simulink model "BG"  (R2014a)
settings: Solver=FixedStepDiscrete  StartTime=0.0  StopTime=24  FixedStep=dt  RelTol=1e-3
values from neighbouring files (symbols this model uses):
  a1 = 5    [parameters.m]
  a2 = 3    [parameters.m]
  a3 = 2    [parameters.m]
  delay = 1    [parameters.m]
  dt = 1e-3    (= 0.001)    [parameters.m]
  g = 1    [parameters.m]
  OP1_0 = [ax1_0 ay1_0 0]    [parameters.m]
  OP2_0 = OP1_0 + P1P2_0    [parameters.m]
  OP3_0 = OP2_0 + P2P3_0    [parameters.m]
  OT1 = [4 6 0]    [animation.m]    (also in parameters.m)
  OT10 = [-1 7.5 0]    [parameters.m]
  OT11 = [3 4.5 0]    [parameters.m]
  OT12 = [-1 7.5 0]    [parameters.m]
  OT2 = [-2 6 0]    [animation.m]    (also in parameters.m)
  OT3 = [1 8 0]    [animation.m]    (also in parameters.m = [4 6 0])
  OT4 = [1 4 0]    [animation.m]    (also in parameters.m = [1 8 0])
  OT5 = [3 7.5 0]    [animation.m]    (also in parameters.m = [1 4 0])
  OT6 = [-1 4.5 0]    [animation.m]    (also in parameters.m = [1 8 0])
  OT7 = [-1 7.5 0]    [animation.m]    (also in parameters.m = [3 7.5 0])
  OT8 = [3 4.5 0]    [animation.m]    (also in parameters.m = [-1 4.5 0])
  OT9 = [3 7.5 0]    [parameters.m]
  P1P2_0 = [ax2_0 ay2_0 0]    [parameters.m]
  P2P3_0 = [ax3_0 ay3_0 0]    [parameters.m]
  w1 = 1/100    (= 0.01)    [parameters.m]
  w2 = 1/50    (= 0.02)    [parameters.m]
  w3 = 1/20    (= 0.05)    [parameters.m]
  zero_vector = [0 0 0]    [parameters.m]
libraries: vrlib x6, simulink x1
settings Model: Creator=Armin  LastModifiedBy=Armin

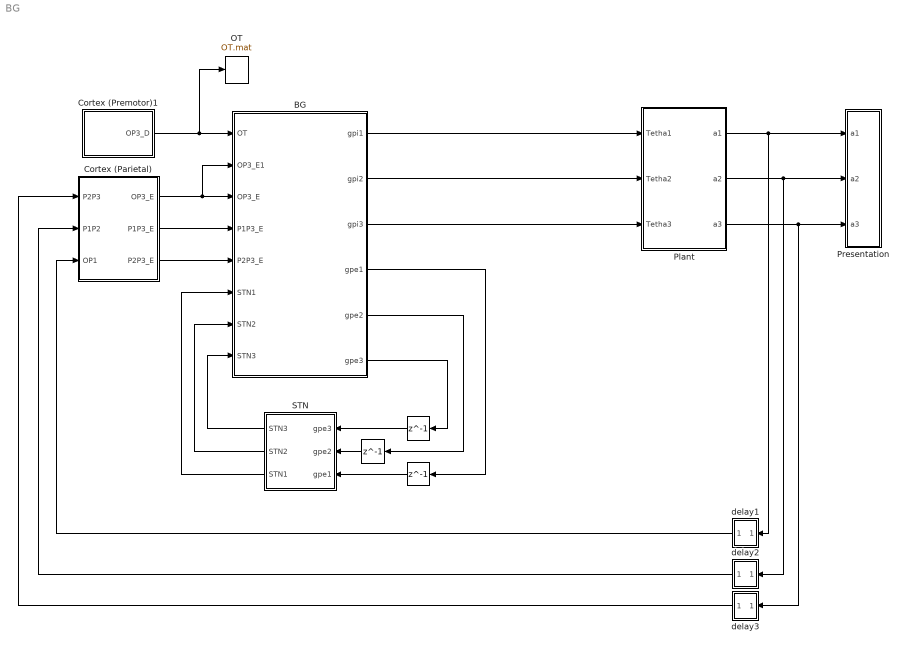
== system BG ==
  "                    " : Delay  DelayLength=1  InitialCondition=zero_vector
  "                     " : Delay  DelayLength=1  InitialCondition=zero_vector
  "                      " : Delay  DelayLength=1  InitialCondition=zero_vector
  BG : Subsystem
  Cortex (Parietal) : Subsystem
  Cortex (Premotor)1 : Subsystem
  OT : ToFile  Filename=OT.mat  MatrixName=T
  Plant : Subsystem
  Presentation : Subsystem
  STN : Subsystem
  delay1 : Subsystem
  delay2 : Subsystem
  delay3 : Subsystem
  wires:
  Plant/1(a1) -> Presentation/1(a1), delay1/1(In1)
  Plant/2(a2) -> Presentation/2(a2), delay2/1(In1)
  BG/1(gpi1) -> Plant/1(Tetha1)
  BG/2(gpi2) -> Plant/2(Tetha2)
  delay2/1(Out1) -> Cortex (Parietal)/2(P1P2)
  delay1/1(Out1) -> Cortex (Parietal)/3(OP1)
  Cortex (Parietal)/1(OP3_E) -> BG/2(OP3_E1), BG/3(OP3_E)
  Cortex (Parietal)/2(P1P3_E) -> BG/4(P1P3_E)
  Cortex (Parietal)/3(P2P3_E) -> BG/5(P2P3_E)
  BG/3(gpi3) -> Plant/3(Tetha3)
  Plant/3(a3) -> Presentation/3(a3), delay3/1(In1)
  delay3/1(Out1) -> Cortex (Parietal)/1(P2P3)
  BG/6(gpe3) -> "                    "/1
  BG/5(gpe2) -> "                     "/1
  BG/4(gpe1) -> "                      "/1
  "                    "/1 -> STN/1(gpe3)
  "                     "/1 -> STN/2(gpe2)
  "                      "/1 -> STN/3(gpe1)
  STN/3(STN1) -> BG/6(STN1)
  STN/2(STN2) -> BG/7(STN2)
  STN/1(STN3) -> BG/8(STN3)
  Cortex (Premotor)1/1(OP3_D) -> OT/1, BG/1(OT)

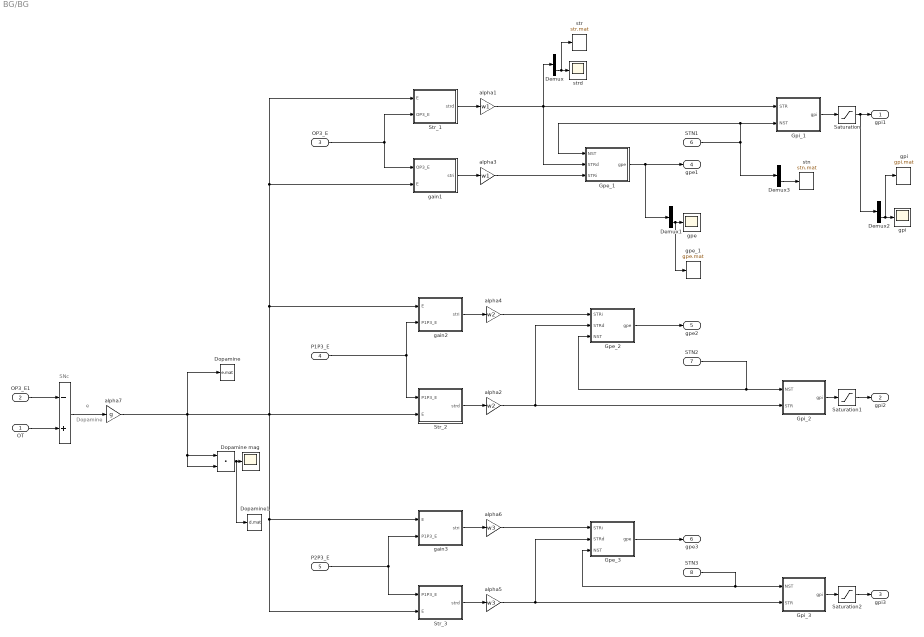
== system BG/BG ==
  note: Dopamine
  note: e
  note: SNc
  OT : Inport
  OP3_E1 : Inport  Port=2
  OP3_E : Inport  Port=3
  P1P3_E : Inport  Port=4
  P2P3_E : Inport  Port=5
  STN1 : Inport  Port=6
  STN2 : Inport  Port=7
  STN3 : Inport  Port=8
  " " : Sum  Inputs=-+
  "     " : DotProduct  InputSameDT=on  OutDataTypeStr=Inherit: Inherit via internal rule
  Demux{,1..3} (4 alike) : Demux  Outputs=3
  Dopamine : ToFile  Filename=e.mat  MatrixName=e
  Dopamine mag : Scope
      settings: SaveName=ScopeData7
  Dopamine1 : ToFile  Filename=d.mat  MatrixName=d
  Gpe_1 : Subsystem
  Gpe_2 : Subsystem
  Gpe_3 : Subsystem
  Gpi_1 : Subsystem
  Gpi_2 : Subsystem
  Gpi_3 : Subsystem
  Saturation : Saturate  UpperLimit=pi  LowerLimit=-pi
  Saturation1 : Saturate  UpperLimit=pi  LowerLimit=-pi
  Saturation2 : Saturate  UpperLimit=pi  LowerLimit=-pi
  Str_1 : Subsystem
  Str_2 : Subsystem
  Str_3 : Subsystem
  alpha1 : Gain  Gain=w1
  alpha2 : Gain  Gain=w2
  alpha3 : Gain  Gain=w1
  alpha4 : Gain  Gain=w2
  alpha5 : Gain  Gain=w3
  alpha6 : Gain  Gain=w3
  alpha7 : Gain  Gain=g
  gain1 : Subsystem
  gain2 : Subsystem
  gain3 : Subsystem
  gpe : Scope
      settings: SaveName=ScopeData5
  gpe_1 : ToFile  Filename=gpe.mat  MatrixName=gpe
  gpi : Scope
      settings: SaveName=ScopeData6
  "gpi " : ToFile  Filename=gpi.mat  MatrixName=gpi
  stn : ToFile  Filename=stn.mat  MatrixName=stn
  str : ToFile  Filename=str.mat  MatrixName=str
  strd : Scope
  gpi1 : Outport
  gpi2 : Outport  Port=2
  gpi3 : Outport  Port=3
  gpe1 : Outport  Port=4
  gpe2 : Outport  Port=5
  gpe3 : Outport  Port=6
  wires:
  Str_1/1(strd) -> alpha1/1
  OP3_E/1 -> gain1/1(OP3_E), Str_1/2(OP3_E)
  Str_2/1(strd) -> alpha2/1
  gain1/1(stri) -> alpha3/1
  alpha3/1 -> Gpe_1/3(STRi)
  Gpe_1/1(gpe) -> Demux1/1, gpe1/1
  STN1/1 -> Demux3/1, Gpi_1/2(NST), Gpe_1/1(NST)
  gain2/1(stri) -> alpha4/1
  alpha4/1 -> Gpe_2/1(STRi)
  P1P3_E/1 -> Str_2/1(P1P3_E), gain2/2(P1P3_E)
  Gpe_2/1(gpe) -> gpe2/1
  OT/1 -> " "/2
  Str_3/1(strd) -> alpha5/1
  gain3/1(stri) -> alpha6/1
  alpha6/1 -> Gpe_3/1(STRi)
  P2P3_E/1 -> Str_3/1(P1P3_E), gain3/2(P1P3_E)
  Gpe_3/1(gpe) -> gpe3/1
  " "/1 -> alpha7/1
  OP3_E1/1 -> " "/1
  Gpi_2/1(gpi) -> Saturation1/1
  Gpi_3/1(gpi) -> Saturation2/1
  Demux/3 -> str/1, strd/1
  Demux1/3 -> gpe_1/1, gpe/1
  Gpi_1/1(gpi) -> Saturation/1
  Demux2/3 -> "gpi "/1, gpi/1
  STN3/1 -> Gpi_3/1(NST), Gpe_3/3(NST)
  STN2/1 -> Gpi_2/1(NST), Gpe_2/3(NST)
  alpha1/1 -> Gpi_1/1(STR), Demux/1, Gpe_1/2(STRd)
  alpha2/1 -> Gpi_2/2(STR), Gpe_2/2(STRd)
  alpha5/1 -> Gpi_3/2(STR), Gpe_3/2(STRd)
  "     "/1 -> Dopamine1/1, Dopamine mag/1
  alpha7/1 -> Str_1/1(E), gain1/2(E), gain2/1(E), Str_2/2(E), gain3/1(E), Str_3/2(E), Dopamine/1, "     "/1, "     "/2
  Saturation/1 -> Demux2/1, gpi1/1
  Saturation1/1 -> gpi2/1
  Saturation2/1 -> gpi3/1
  Demux3/3 -> stn/1

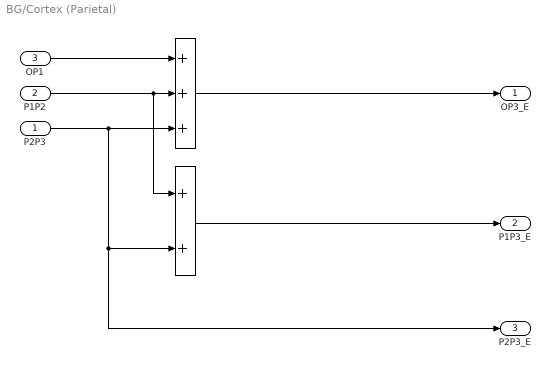
== system BG/Cortex (Parietal) ==
  P2P3 : Inport
  P1P2 : Inport  Port=2
  OP1 : Inport  Port=3
  " " : Sum  Inputs=+++
  "  " : Sum
  OP3_E : Outport
  P1P3_E : Outport  Port=2
  P2P3_E : Outport  Port=3
  wires:
  OP1/1 -> " "/1
  P1P2/1 -> "  "/1, " "/2
  P2P3/1 -> P2P3_E/1, "  "/2, " "/3
  " "/1 -> OP3_E/1
  "  "/1 -> P1P3_E/1

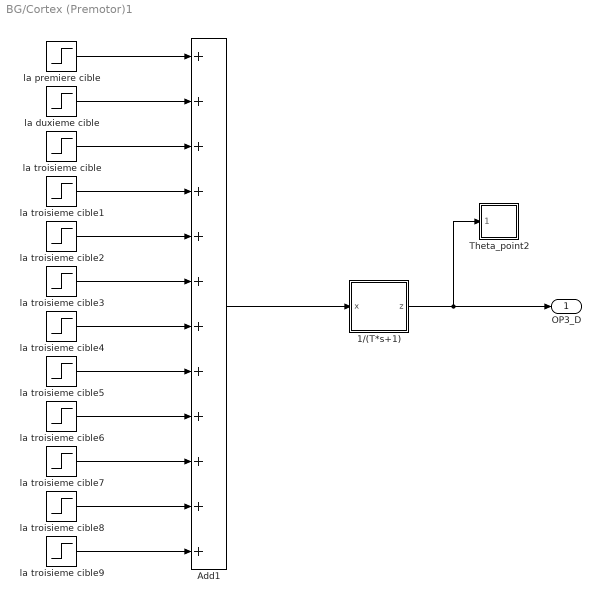
== system BG/Cortex (Premotor)1 ==
  1/(T*s+1) : Subsystem  TreatAsAtomicUnit=on
  Add1 : Sum  Inputs=++++++++++++
  Theta_point2 : Subsystem
  la duxieme cible : Step  Time=2  After=OT2-OT1  SampleTime=0
  la premiere cible : Step  Time=0.05  Before=OP3_0  After=OT1  SampleTime=0
  la troisieme cible : Step  Time=4  After=OT3-OT2  SampleTime=0
  la troisieme cible1 : Step  Time=6  After=OT4-OT3  SampleTime=0
  la troisieme cible2 : Step  Time=8  After=OT5-OT4  SampleTime=0
  la troisieme cible3 : Step  Time=10  After=OT6-OT5  SampleTime=0
  la troisieme cible4 : Step  Time=12  After=OT7-OT6  SampleTime=0
  la troisieme cible5 : Step  Time=14  After=OT8-OT7  SampleTime=0
  la troisieme cible6 : Step  Time=16  After=OT9-OT8  SampleTime=0
  la troisieme cible7 : Step  Time=18  After=OT10-OT9  SampleTime=0
  la troisieme cible8 : Step  Time=20  After=OT11-OT10  SampleTime=0
  la troisieme cible9 : Step  Time=22  After=OT12-OT11  SampleTime=0
  OP3_D : Outport
  wires:
  1/(T*s+1)/1(z) -> Theta_point2/1(In_vec), OP3_D/1
  Add1/1 -> 1/(T*s+1)/1(x)
  la premiere cible/1 -> Add1/1
  la duxieme cible/1 -> Add1/2
  la troisieme cible/1 -> Add1/3
  la troisieme cible1/1 -> Add1/4
  la troisieme cible2/1 -> Add1/5
  la troisieme cible3/1 -> Add1/6
  la troisieme cible4/1 -> Add1/7
  la troisieme cible5/1 -> Add1/8
  la troisieme cible6/1 -> Add1/9
  la troisieme cible7/1 -> Add1/10
  la troisieme cible8/1 -> Add1/11
  la troisieme cible9/1 -> Add1/12

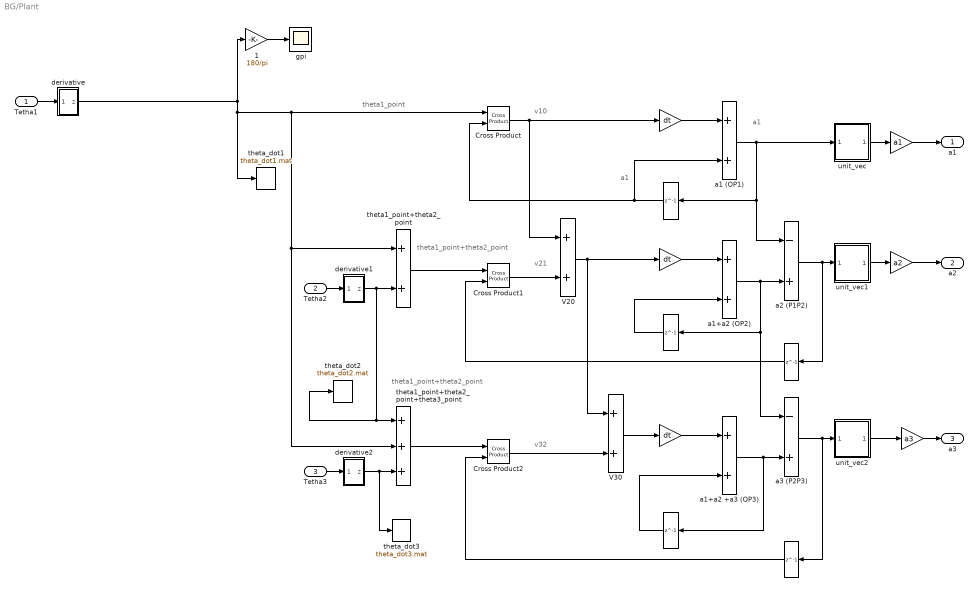
== system BG/Plant ==
  note: theta1_point
  note: a1
  note: v10
  note: a1
  note: theta1_point+theta2_point
  note: v21
  note: theta1_point+theta2_point
  note: v32
  Tetha1 : Inport
  Tetha2 : Inport  Port=2
  Tetha3 : Inport  Port=3
  " " : Delay  DelayLength=1  InitialCondition=OP1_0
  "  " : Delay  DelayLength=1  InitialCondition=OP2_0
  "        " : Gain  Gain=dt
  "         " : Gain  Gain=a1
  "          " : Delay  DelayLength=1  InitialCondition=OP3_0
  "              " : Gain  Gain=a2
  "                  " : Delay  DelayLength=1  InitialCondition=P1P2_0
  "                         " : Gain  Gain=a3
  "                                  " : Gain  Gain=dt
  "                                                             " : Gain  Gain=dt
  "                                                              " : Delay  DelayLength=1  InitialCondition=P2P3_0
  "        1" : Gain  Gain=180/pi
  "Cross Product " : vrlib/Utilities/Cross Product
  Cross Product1 : vrlib/Utilities/Cross Product
  Cross Product2 : vrlib/Utilities/Cross Product
  V20 : Sum
  V30 : Sum
  a1 (OP1) : Sum
  a1+a2 (OP2) : Sum
  a1+a2 +a3 (OP3) : Sum
  a2 (P1P2) : Sum  Inputs=-+
  a3 (P2P3) : Sum  Inputs=-+
  derivative : Subsystem  TreatAsAtomicUnit=on
  derivative1 : Subsystem  TreatAsAtomicUnit=on
  derivative2 : Subsystem  TreatAsAtomicUnit=on
  gpi : Scope
      settings: YMin=-6.5e-35  YMax=0  SaveName=ScopeData8
  theta1_point+theta2_point : Sum
  theta1_point+theta2_point+theta3_point : Sum  Inputs=+++
  theta_dot1 : ToFile  Filename=theta_dot1.mat  MatrixName=theta_dot1
  theta_dot2 : ToFile  Filename=theta_dot2.mat  MatrixName=theta_dot2
  theta_dot3 : ToFile  Filename=theta_dot3.mat  MatrixName=theta_dot3
  unit_vec : Subsystem
  unit_vec1 : Subsystem
  unit_vec2 : Subsystem
  a1 : Outport
  a2 : Outport  Port=2
  a3 : Outport  Port=3
  wires:
  "        "/1 -> a1 (OP1)/1
  " "/1 -> "Cross Product "/2, a1 (OP1)/2
  Tetha1/1 -> derivative/1(x)
  Tetha2/1 -> derivative1/1(x)
  theta1_point+theta2_point/1 -> Cross Product1/1
  Tetha3/1 -> derivative2/1(x)
  theta1_point+theta2_point+theta3_point/1 -> Cross Product2/1
  V20/1 -> "                                  "/1, V30/1
  "                                  "/1 -> a1+a2 (OP2)/1
  a1+a2 (OP2)/1 -> a2 (P1P2)/2, a3 (P2P3)/1, "  "/1
  "  "/1 -> a1+a2 (OP2)/2
  "                  "/1 -> Cross Product1/2
  V30/1 -> "                                                             "/1
  a1+a2 +a3 (OP3)/1 -> a3 (P2P3)/2, "          "/1
  "          "/1 -> a1+a2 +a3 (OP3)/2
  "                                                              "/1 -> Cross Product2/2
  "                                                             "/1 -> a1+a2 +a3 (OP3)/1
  "Cross Product "/1 -> V20/1, "        "/1
  Cross Product1/1 -> V20/2
  Cross Product2/1 -> V30/2
  a1 (OP1)/1 -> a2 (P1P2)/1, " "/1, unit_vec/1(vec1)
  a2 (P1P2)/1 -> "                  "/1, unit_vec1/1(vec1)
  a3 (P2P3)/1 -> unit_vec2/1(vec1), "                                                              "/1
  unit_vec/1(vec2) -> "         "/1
  "         "/1 -> a1/1
  unit_vec1/1(vec2) -> "              "/1
  "              "/1 -> a2/1
  "                         "/1 -> a3/1
  unit_vec2/1(vec2) -> "                         "/1
  derivative1/1(z) -> theta_dot2/1, theta1_point+theta2_point+theta3_point/1, theta1_point+theta2_point/2
  derivative2/1(z) -> theta_dot3/1, theta1_point+theta2_point+theta3_point/3
  "        1"/1 -> gpi/1
  derivative/1(z) -> theta_dot1/1, "Cross Product "/1, theta1_point+theta2_point/1, theta1_point+theta2_point+theta3_point/2, "        1"/1

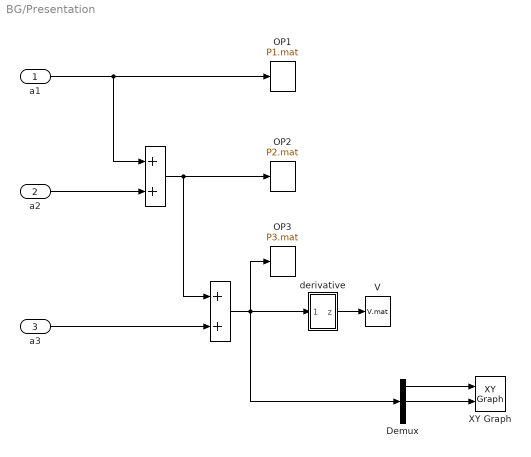
== system BG/Presentation ==
  a1 : Inport
  a2 : Inport  Port=2
  a3 : Inport  Port=3
  "                       " : Sum
  "                        " : Sum
  Demux : Demux  Outputs=3
  OP1 : ToFile  Filename=P1.mat  MatrixName=P1
  OP2 : ToFile  Filename=P2.mat  MatrixName=P2
  OP3 : ToFile  Filename=P3.mat  MatrixName=P3
  V : ToFile  Filename=V.mat  MatrixName=V
  XY Graph : simulink/Sinks/XY Graph  xmin=-10  xmax=10  ymin=0  ymax=10  st=-1
  derivative : Subsystem  TreatAsAtomicUnit=on
  wires:
  a1/1 -> "                       "/1, OP1/1
  a2/1 -> "                       "/2
  "                       "/1 -> "                        "/1, OP2/1
  a3/1 -> "                        "/2
  "                        "/1 -> Demux/1, OP3/1, derivative/1(x)
  derivative/1(z) -> V/1
  Demux/1 -> XY Graph/1
  Demux/2 -> XY Graph/2

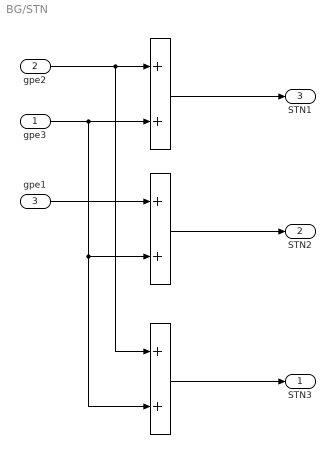
== system BG/STN ==
  gpe3 : Inport
  gpe2 : Inport  Port=2
  gpe1 : Inport  Port=3
  " " : Sum
  "  " : Sum
  "    " : Sum
  STN3 : Outport
  STN2 : Outport  Port=2
  STN1 : Outport  Port=3
  wires:
  " "/1 -> STN1/1
  gpe3/1 -> " "/2, "    "/2, "  "/2
  gpe2/1 -> " "/1, "    "/1
  "  "/1 -> STN2/1
  gpe1/1 -> "  "/1
  "    "/1 -> STN3/1

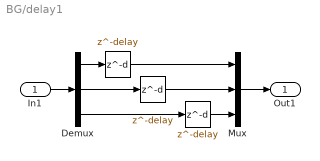
== system BG/delay1 ==
  In1 : Inport
  "  " : Delay  DelayLength=delay  InitialCondition=OP1_0(2)
  "   " : Delay  DelayLength=delay  InitialCondition=OP1_0(3)
  "                                                                                                                                               \t" : Delay  DelayLength=delay  InitialCondition=OP1_0(1)
  Demux : Demux  Outputs=3
  Mux : Mux  Inputs=3
  Out1 : Outport
  wires:
  Mux/1 -> Out1/1
  In1/1 -> Demux/1
  "                                                                                                                                               \t"/1 -> Mux/1
  Demux/1 -> "                                                                                                                                               \t"/1
  "  "/1 -> Mux/2
  Demux/2 -> "  "/1
  "   "/1 -> Mux/3
  Demux/3 -> "   "/1

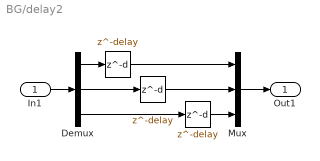
== system BG/delay2 ==
  In1 : Inport
  "  " : Delay  DelayLength=delay  InitialCondition=P1P2_0(2)
  "   " : Delay  DelayLength=delay  InitialCondition=P1P2_0(3)
  "                                                                                                                                               \t" : Delay  DelayLength=delay  InitialCondition=P1P2_0(1)
  Demux : Demux  Outputs=3
  Mux : Mux  Inputs=3
  Out1 : Outport
  wires:
  Mux/1 -> Out1/1
  In1/1 -> Demux/1
  "                                                                                                                                               \t"/1 -> Mux/1
  Demux/1 -> "                                                                                                                                               \t"/1
  "  "/1 -> Mux/2
  Demux/2 -> "  "/1
  "   "/1 -> Mux/3
  Demux/3 -> "   "/1

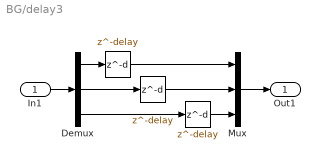
== system BG/delay3 ==
  In1 : Inport
  "  " : Delay  DelayLength=delay  InitialCondition=P2P3_0(2)
  "   " : Delay  DelayLength=delay  InitialCondition=P2P3_0(3)
  "                                                                                                                                               \t" : Delay  DelayLength=delay  InitialCondition=P2P3_0(1)
  Demux : Demux  Outputs=3
  Mux : Mux  Inputs=3
  Out1 : Outport
  wires:
  Mux/1 -> Out1/1
  In1/1 -> Demux/1
  "                                                                                                                                               \t"/1 -> Mux/1
  Demux/1 -> "                                                                                                                                               \t"/1
  "  "/1 -> Mux/2
  Demux/2 -> "  "/1
  "   "/1 -> Mux/3
  Demux/3 -> "   "/1

== system BG/BG/Gpe_1 ==
  NST : Inport
  STRd : Inport  Port=2
  STRi : Inport  Port=3
  "   " : Product
  GPi1 : Sum  Inputs=+-
  gpe : Outport
  wires:
  STRd/1 -> GPi1/1
  NST/1 -> GPi1/2
  GPi1/1 -> "   "/1
  STRi/1 -> "   "/2
  "   "/1 -> gpe/1

== system BG/BG/Gpe_2 ==
  STRi : Inport
  STRd : Inport  Port=2
  NST : Inport  Port=3
  "   " : Product
  GPi1 : Sum  Inputs=+-
  gpe : Outport
  wires:
  STRd/1 -> GPi1/1
  NST/1 -> GPi1/2
  GPi1/1 -> "   "/1
  STRi/1 -> "   "/2
  "   "/1 -> gpe/1

== system BG/BG/Gpe_3 ==
  STRi : Inport
  STRd : Inport  Port=2
  NST : Inport  Port=3
  "   " : Product
  GPi1 : Sum  Inputs=+-
  gpe : Outport
  wires:
  STRd/1 -> GPi1/1
  NST/1 -> GPi1/2
  GPi1/1 -> "   "/1
  STRi/1 -> "   "/2
  "   "/1 -> gpe/1

== system BG/BG/Gpi_1 ==
  STR : Inport
  NST : Inport  Port=2
  "                  " : Delay  DelayLength=1  InitialCondition=zero_vector
  GPi1 : Sum  Inputs=++-
  gpi : Outport
  wires:
  GPi1/1 -> "                  "/1, gpi/1
  "                  "/1 -> GPi1/1
  STR/1 -> GPi1/2
  NST/1 -> GPi1/3

== system BG/BG/Gpi_2 ==
  NST : Inport
  STR : Inport  Port=2
  "                  " : Delay  DelayLength=1  InitialCondition=zero_vector
  GPi1 : Sum  Inputs=++-
  gpi : Outport
  wires:
  GPi1/1 -> "                  "/1, gpi/1
  "                  "/1 -> GPi1/1
  STR/1 -> GPi1/2
  NST/1 -> GPi1/3

== system BG/BG/Gpi_3 ==
  NST : Inport
  STR : Inport  Port=2
  "                  " : Delay  DelayLength=1  InitialCondition=zero_vector
  GPi1 : Sum  Inputs=++-
  gpi : Outport
  wires:
  GPi1/1 -> "                  "/1, gpi/1
  "                  "/1 -> GPi1/1
  STR/1 -> GPi1/2
  NST/1 -> GPi1/3

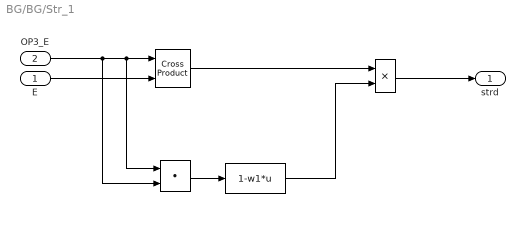
== system BG/BG/Str_1 ==
  E : Inport
  OP3_E : Inport  Port=2
  "  " : Fcn  Expr=1-w1*u
  "   " : Product
  "    " : DotProduct  InputSameDT=on  OutDataTypeStr=Inherit: Inherit via internal rule
  "       " : vrlib/Utilities/Cross Product
  strd : Outport
  wires:
  OP3_E/1 -> "    "/2, "    "/1, "       "/1
  E/1 -> "       "/2
  "    "/1 -> "  "/1
  "       "/1 -> "   "/1
  "  "/1 -> "   "/2
  "   "/1 -> strd/1

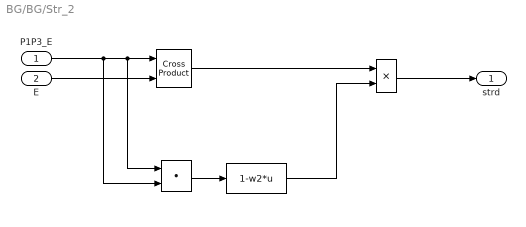
== system BG/BG/Str_2 ==
  P1P3_E : Inport
  E : Inport  Port=2
  "  " : Fcn  Expr=1-w2*u
  "   " : Product
  "    " : DotProduct  InputSameDT=on  OutDataTypeStr=Inherit: Inherit via internal rule
  "       " : vrlib/Utilities/Cross Product
  strd : Outport
  wires:
  P1P3_E/1 -> "    "/2, "    "/1, "       "/1
  E/1 -> "       "/2
  "    "/1 -> "  "/1
  "       "/1 -> "   "/1
  "  "/1 -> "   "/2
  "   "/1 -> strd/1

== system BG/BG/Str_3 ==
  P1P3_E : Inport
  E : Inport  Port=2
  "  " : Fcn  Expr=1-w3*u
  "   " : Product
  "    " : DotProduct  InputSameDT=on  OutDataTypeStr=Inherit: Inherit via internal rule
  "       " : vrlib/Utilities/Cross Product
  strd : Outport
  wires:
  P1P3_E/1 -> "    "/2, "    "/1, "       "/1
  E/1 -> "       "/2
  "    "/1 -> "  "/1
  "       "/1 -> "   "/1
  "  "/1 -> "   "/2
  "   "/1 -> strd/1

== system BG/BG/gain1 ==
  OP3_E : Inport
  E : Inport  Port=2
  "     " : DotProduct  InputSameDT=on  OutDataTypeStr=Inherit: Inherit via internal rule
  stri : Outport
  wires:
  OP3_E/1 -> "     "/1
  E/1 -> "     "/2
  "     "/1 -> stri/1

== system BG/BG/gain2 ==
  E : Inport
  P1P3_E : Inport  Port=2
  "     " : DotProduct  InputSameDT=on  OutDataTypeStr=Inherit: Inherit via internal rule
  stri : Outport
  wires:
  P1P3_E/1 -> "     "/1
  E/1 -> "     "/2
  "     "/1 -> stri/1

== system BG/BG/gain3 ==
  E : Inport
  P1P3_E : Inport  Port=2
  "     " : DotProduct  InputSameDT=on  OutDataTypeStr=Inherit: Inherit via internal rule
  stri : Outport
  wires:
  P1P3_E/1 -> "     "/1
  E/1 -> "     "/2
  "     "/1 -> stri/1

== system BG/Cortex (Premotor)1/1//(T*s+1) ==
  x : Inport
  Add : Sum  Inputs=+-
  Add1 : Sum
  Delay : Delay  DelayLength=1  InitialCondition=OP3_0
  Gain : Gain  Gain=dt
  Gain2 : Gain  Gain=1/0.05
  z : Outport
  wires:
  Add/1 -> Gain/1
  Delay/1 -> Add1/2, Add/2
  Gain/1 -> Gain2/1
  x/1 -> Add/1
  Add1/1 -> z/1, Delay/1
  Gain2/1 -> Add1/1

== system BG/Cortex (Premotor)1/Theta_point2 ==
  In_vec : Inport
  Demux : Demux  Outputs=3
  x : Scope
  y : Scope
      settings: SaveName=ScopeData2
  z : Scope
      settings: SaveName=ScopeData3
  wires:
  In_vec/1 -> Demux/1
  Demux/1 -> x/1
  Demux/2 -> y/1
  Demux/3 -> z/1

== system BG/Plant/derivative ==
  x : Inport
  Add : Sum  Inputs=+-
  Delay : Delay  DelayLength=1  InitialCondition=zero_vector
  Gain : Gain  Gain=1/dt
  z : Outport
  wires:
  Add/1 -> Gain/1
  x/1 -> Delay/1, Add/1
  Delay/1 -> Add/2
  Gain/1 -> z/1

== system BG/Plant/derivative1 ==
  x : Inport
  Add : Sum  Inputs=+-
  Delay : Delay  DelayLength=1  InitialCondition=zero_vector
  Gain : Gain  Gain=1/dt
  z : Outport
  wires:
  Add/1 -> Gain/1
  x/1 -> Delay/1, Add/1
  Delay/1 -> Add/2
  Gain/1 -> z/1

== system BG/Plant/derivative2 ==
  x : Inport
  Add : Sum  Inputs=+-
  Delay : Delay  DelayLength=1  InitialCondition=zero_vector
  Gain : Gain  Gain=1/dt
  z : Outport
  wires:
  Add/1 -> Gain/1
  x/1 -> Delay/1, Add/1
  Delay/1 -> Add/2
  Gain/1 -> z/1

== system BG/Plant/unit_vec ==
  vec1 : Inport
  Divide : Product  Inputs=*/
  Dot Product3 : DotProduct  InputSameDT=on  OutDataTypeStr=Inherit: Inherit via internal rule
  Sqrt : Sqrt  SaturateOnIntegerOverflow=on
  vec2 : Outport
  wires:
  vec1/1 -> Divide/1, Dot Product3/2, Dot Product3/1
  Dot Product3/1 -> Sqrt/1
  Sqrt/1 -> Divide/2
  Divide/1 -> vec2/1

== system BG/Plant/unit_vec1 ==
  vec1 : Inport
  Divide : Product  Inputs=*/
  Dot Product3 : DotProduct  InputSameDT=on  OutDataTypeStr=Inherit: Inherit via internal rule
  Sqrt : Sqrt  SaturateOnIntegerOverflow=on
  vec2 : Outport
  wires:
  vec1/1 -> Divide/1, Dot Product3/2, Dot Product3/1
  Dot Product3/1 -> Sqrt/1
  Sqrt/1 -> Divide/2
  Divide/1 -> vec2/1

== system BG/Plant/unit_vec2 ==
  vec1 : Inport
  Divide : Product  Inputs=*/
  Dot Product3 : DotProduct  InputSameDT=on  OutDataTypeStr=Inherit: Inherit via internal rule
  Sqrt : Sqrt  SaturateOnIntegerOverflow=on
  vec2 : Outport
  wires:
  vec1/1 -> Divide/1, Dot Product3/2, Dot Product3/1
  Dot Product3/1 -> Sqrt/1
  Sqrt/1 -> Divide/2
  Divide/1 -> vec2/1

== system BG/Presentation/derivative ==
  x : Inport
  Add : Sum  Inputs=+-
  Delay : Delay  DelayLength=1  InitialCondition=OP3_0
  Gain : Gain  Gain=1/dt
  z : Outport
  wires:
  Add/1 -> Gain/1
  x/1 -> Delay/1, Add/1
  Delay/1 -> Add/2
  Gain/1 -> z/1
